simulink model "fm_cw_radar_system"  (Simulink 7.5)
settings: Solver=ode45  StartTime=0.0  StopTime=20  RelTol=1e-3
undefined symbols (not defined in the file): Fs, get, sided, Two
libraries: dsparch4 x1, commsynccomp2 x1, simulink x1, commnoisgen2 x1, dspsnks4 x1
settings Model: Creator=LG  LastModifiedBy=mohamed alasklany
settings SimEventsCC: propDiagAttribOutput=1  propDiagFcnCallOutput=1  propDiagStatOutput=0

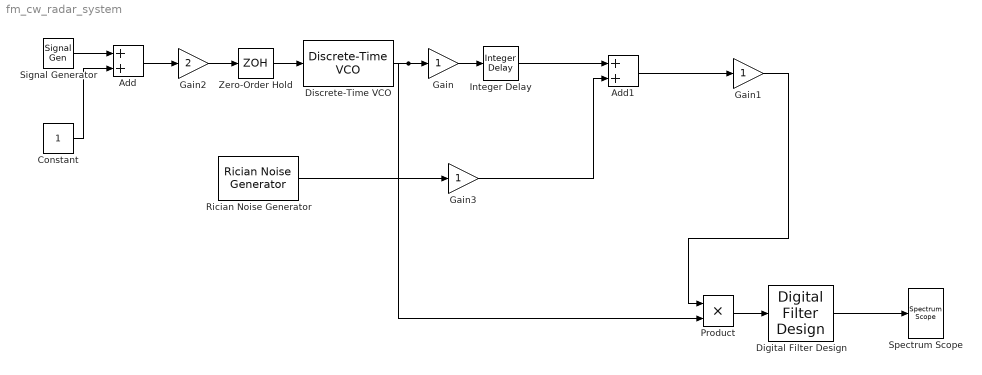
== system fm_cw_radar_system ==
  Add : Sum  OutDataType=fixdt(1, 16)  OutScaling=2^-10
  Add1 : Sum  OutDataType=fixdt(1, 16)  OutScaling=2^-10
  Constant : Constant  OutDataType=fixdt(1, 16)  OutScaling=2^0
  Digital Filter Design : dsparch4/Digital Filter Design  SystemSampleTime=-1  mwdsp_browser_bugfix_var=off
  Discrete-Time VCO : commsynccomp2/Discrete-Time VCO  SystemSampleTime=-1  Ac=1  Fc=1e5  Kc=10000  Ph=0  ts=1/(2.08e6)
  Gain : Gain  ParameterDataType=fixdt(1, 16)  ParameterScaling=2^0  OutDataType=fixdt(1, 16)  OutScaling=2^0
  Gain1 : Gain  ParameterDataType=fixdt(1, 16)  ParameterScaling=2^0  OutDataType=fixdt(1, 16)  OutScaling=2^0
  Gain2 : Gain  Gain=2  ParameterDataType=fixdt(1, 16)  ParameterScaling=2^0  OutDataType=fixdt(1, 16)  OutScaling=2^0
  Gain3 : Gain  ParameterDataType=fixdt(1, 16)  ParameterScaling=2^0  OutDataType=fixdt(1, 16)  OutScaling=2^0
  Integer Delay : simulink/Discrete/Integer Delay  vinit=0.0  samptime=-1  NumDelays=6000
  Product : Product  OutDataType=fixdt(1, 16)  OutScaling=2^0  RndMeth=Zero
  Rician Noise Generator : commnoisgen2/Rician Noise Generator  SystemSampleTime=-1  specMethod=K-factor  iMean=sqrt(2)  qMean=sqrt(2)  K=2  s=2  seed=10  Ts=1/2.08e6  frameBased=off  sampPerFrame=1  orient=on  outDataType=double
  Signal Generator : SignalGenerator  WaveForm=sawtooth  Frequency=1000
  Spectrum Scope : dspsnks4/Spectrum Scope  DialogController=dspdialog.SpectrumScope  DialogControllerArgs=DataTag1  SystemSampleTime=-1  ScopeProperties=on  Domain=Frequency  HorizSpan=1  UseBuffer=on  BufferSize=4*2048  Overlap=1024  inpFftLenInherit=off  FFTlength=256  numAvg=2  DisplayProperties=off  AxisGrid=on  Memory=off  FrameNumber=on  AxisLegend=off  AxisZoom=off  OpenScopeAtSimStart=on  OpenScopeImmediately=off  FigPos=get(0,'defaultfigureposition')  AxisProperties=off  XUnits=Hertz  XRange=Two-sided ((-Fs/2...Fs/2])  XDisplay=0  InheritXIncr=on  XIncr=1/1e9  XLabel=Samples  XLimit=User-defined  YUnits=dBm  XMax=10000  XMin=-10000  YLabel=Magnitude-squared, dBm  LineProperties=off  wintypeSpecScope=Hamming  RsSpecScope=50  betaSpecScope=5  winsampSpecScope=Periodic  XAxisParamsVer=6.9
      settings: YMin=-10  YMax=50
  Zero-Order Hold : ZeroOrderHold  SampleTime=1/(2.08e6)
  wires:
  Discrete-Time VCO/1 -> Gain/1, Product/2
  Gain/1 -> Integer Delay/1
  Gain1/1 -> Product/1
  Zero-Order Hold/1 -> Discrete-Time VCO/1
  Signal Generator/1 -> Add/1
  Constant/1 -> Add/2
  Add/1 -> Gain2/1
  Gain2/1 -> Zero-Order Hold/1
  Product/1 -> Digital Filter Design/1
  Digital Filter Design/1 -> Spectrum Scope/1
  Rician Noise Generator/1 -> Gain3/1
  Add1/1 -> Gain1/1
  Integer Delay/1 -> Add1/1
  Gain3/1 -> Add1/2
